simulink model "statefdbk_integral"  (R2023a)
settings: Solver=ode45  StartTime=0.0  StopTime=20  RelTol=1e-3
values from neighbouring files (symbols this model uses):
  A = [A zeros(n,1); -C_ 1]    [control_integral.m]    (also in model.mat = [2.19826062055 1 0 0 0 0 -0.950981109251 0 1 0 0 0 ... (36 e; square_2V_2_5hz_100fs.mat = [3.68944323306 1 0 0 0 0 0 0 0 0 0 -4.87835143564 ... (121 e; square_2V_2_5hz_50fs.mat = [3.32314178319 1 0 0 0 0 0 0 0 0 0 -4.05203564565 ... (121 e)
  B = [B ; 0]    [control_integral.m]    (also in model.mat = [1 0 0 0 0 0]; square_2V_2_5hz_100fs.mat = [1 0 0 0 0 0 0 0 0 0 0]; square_2V_2_5hz_50fs.mat = [1 0 0 0 0 0 0 0 0 0 0])
  C = eye(6)    [control.m]    (also in control_integral.m; model.mat = [-0.0688244704241 0.243744146338 -0.160379964746 0.159733475; square_2V_2_5hz_100fs.mat = [0.0387406639515 -0.00769875135999 -0.0877071898369 0.106733; square_2V_2_5hz_50fs.mat = [0.137657900871 -0.107456657028 -0.0846958769464 0.059459958)
  C_ = C    [control.m]    (also in control_integral.m)
  D = zeros(size(A,1),1)    [control.m]    (also in control_integral.m; model.mat = 0; plotter.m = sign(tensao_gage.signals.values(2))*str2double(strcat(newStr; square_2V_2_5hz_100fs.mat = 0)
  K = dlqr(A,B,Q,R)    [control.m]    (also in control_integral.m = K(1:end-1))
  Ki = K(end)    [control_integral.m]
  L = dlqe(A,G,C,Q_w,R_v)    [control.m]    (also in control_integral.m; plotter.m = convlength(L,'in','m')*100)
  x0 = [0 0 0 0 0 10]    [control.m]    (also in control_integral.m = [0 0 0 0 0 0]; model_identification_ecpd.m = findstates(sys,iddata(y,u,1/fs)))
settings Model: Creator=Tiago  LastModifiedBy=Tiago
settings SolverCC: AlgebraicLoopSolver=TrustRegion
settings DataIOCC: ReturnWorkspaceOutputs=off
settings OptimizationCC: LifeSpan=inf
settings DebuggingCC: UnconnectedInputMsg=warning  UnconnectedOutputMsg=warning  UnconnectedLineMsg=warning  SFExecutionAtInitializationDiag=none  ArithmeticOperatorsInVariantConditions=warning
settings HardwareCC: ProdBitPerSizeT=32  ProdBitPerPtrDiffT=32  ProdWordSize=32  ProdHWDeviceType=Specified
settings SFSimCC: CustomCodeUndefinedFunction=UseInterfaceOnly
settings CodeAppCC: StateflowObjectComments=on

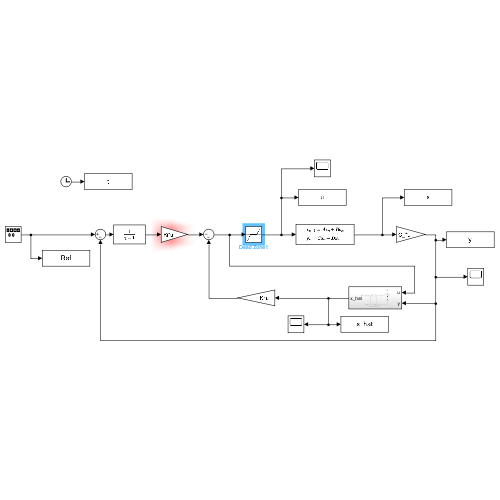
[thumbnail: Simulink's stored preview of the top-level diagram]
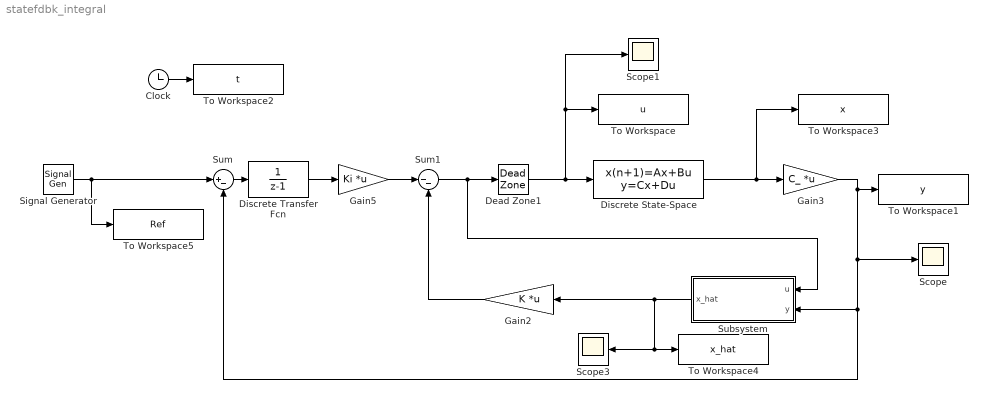
== system statefdbk_integral ==
  Clock : Clock
  Dead Zone1 : DeadZone  LowerValue=-0.3  UpperValue=0.3
  Discrete Transfer Fcn : DiscreteTransferFcn  Denominator=[1 -1]
  Discrete State-Space : DiscreteStateSpace  A=A  B=B  C=C  D=D  InitialCondition=x0  SampleTime=0.02
  Gain2 : Gain  Gain=K  Multiplication=Matrix(K*u)
  Gain3 : Gain  Gain=C_  Multiplication=Matrix(K*u)
  Gain5 : Gain  Gain=Ki  Multiplication=Matrix(K*u)
  Scope : Scope
  Scope1 : Scope
  Scope3 : Scope
  Signal Generator : SignalGenerator  WaveForm=square  Amplitude=20  Frequency=0.5
  Subsystem : Subsystem
  Sum : Sum  Inputs=|+-
  Sum1 : Sum  Inputs=|--
  To Workspace : ToWorkspace  VariableName=u  SaveFormat=Structure With Time  SampleTime=0.02
  To Workspace1 : ToWorkspace  VariableName=y  SaveFormat=Structure With Time  SampleTime=0.02
  To Workspace2 : ToWorkspace  VariableName=t  SampleTime=0.02
  To Workspace3 : ToWorkspace  VariableName=x  SaveFormat=Structure With Time  SampleTime=-1
  To Workspace4 : ToWorkspace  VariableName=x_hat  SaveFormat=Structure With Time  SampleTime=0.02
  To Workspace5 : ToWorkspace  VariableName=Ref  SaveFormat=Structure With Time  SampleTime=-1
  wires:
  Discrete State-Space/1 -> Gain3/1, To Workspace3/1
  Subsystem/1(x_hat) -> Scope3/1, To Workspace4/1, Gain2/1
  Signal Generator/1 -> Sum/1, To Workspace5/1
  Dead Zone1/1 -> Discrete State-Space/1, Scope1/1, To Workspace/1
  Clock/1 -> To Workspace2/1
  Gain2/1 -> Sum1/2
  Sum1/1 -> Subsystem/1(u), Dead Zone1/1
  Gain3/1 -> Sum/2, Subsystem/2(y), Scope/1, To Workspace1/1
  Gain5/1 -> Sum1/1
  Sum/1 -> Discrete Transfer Fcn/1
  Discrete Transfer Fcn/1 -> Gain5/1

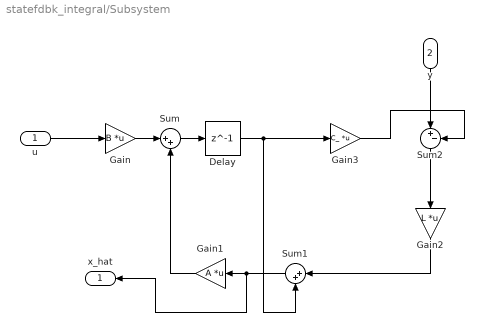
== system statefdbk_integral/Subsystem ==
  u : Inport
  y : Inport  Port=2
  Delay : Delay  DelayLength=1  InitialCondition=0
  Gain : Gain  Gain=B  Multiplication=Matrix(K*u)
  Gain1 : Gain  Gain=A  Multiplication=Matrix(K*u)
  Gain2 : Gain  Gain=L  Multiplication=Matrix(K*u)
  Gain3 : Gain  Gain=C_  Multiplication=Matrix(K*u)
  Sum : Sum  Inputs=|++
  Sum1 : Sum  Inputs=|++
  Sum2 : Sum  Inputs=|+-
  x_hat : Outport
  wires:
  u/1 -> Gain/1
  Gain3/1 -> Sum2/2
  y/1 -> Sum2/1
  Sum2/1 -> Gain2/1
  Gain2/1 -> Sum1/1
  Delay/1 -> Gain3/1, Sum1/2
  Sum1/1 -> x_hat/1, Gain1/1
  Gain/1 -> Sum/1
  Sum/1 -> Delay/1
  Gain1/1 -> Sum/2
